simulink model "TrafficLightControl"  (R2020b)
settings: Solver=FixedStepDiscrete  StartTime=0.0  StopTime=150  FixedStep=0.1  RelTol=1e-3  EnableMultiTasking=on
undefined symbols (not defined in the file): DiscIntNeverNeededParam
libraries: simulink x1
settings Model: Creator=baner  LastModifiedBy=baner
settings DataIOCC: ReturnWorkspaceOutputs=off
settings HardwareCC: ProdHWDeviceType=AMD->x86-64 (Windows64)
settings SFSimCC: SimParseCustomCode=off

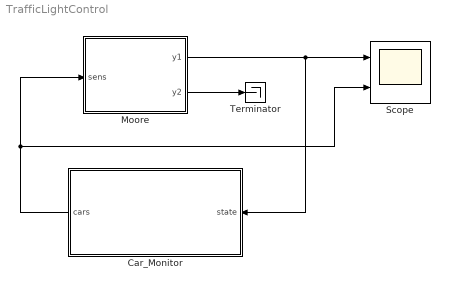
== system TrafficLightControl ==
  Car_Monitor : Subsystem
  Moore : Stateflow chart  TreatAsAtomicUnit=on
  Scope : Scope  NumInputPorts=2
  Terminator : Terminator
  wires:
  Moore/1(y1) -> Car_Monitor/1(state), Scope/1
  Car_Monitor/1(cars) -> Moore/1(sens), Scope/2
  Moore/2(y2) -> Terminator/1

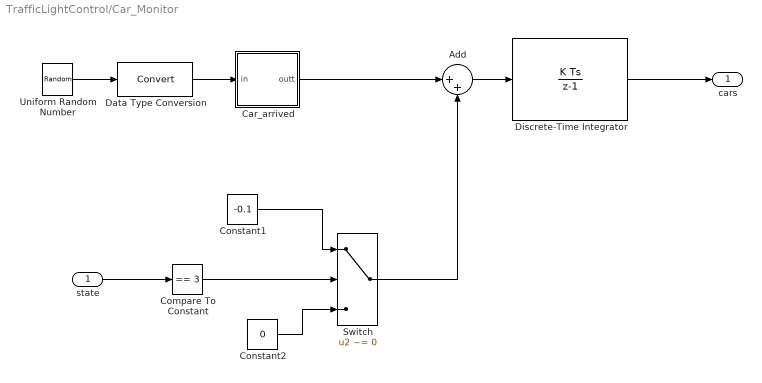
== system TrafficLightControl/Car_Monitor ==
  state : Inport
  Add : Sum  Inputs=|++
  Car_arrived : Stateflow chart  TreatAsAtomicUnit=on
  Compare To Constant : simulink/Logic and Bit Operations/Compare To Constant  relop===  const=3  OutDataTypeStr=boolean  ZeroCross=off
  Constant1 : Constant  Value=-0.1
  Constant2 : Constant  Value=0
  Data Type Conversion : DataTypeConversion
  Discrete-Time Integrator : DiscreteIntegrator  SampleTime=-1  LimitOutput=on  LowerSaturationLimit=0  ICPrevOutput=DiscIntNeverNeededParam  ICPrevScaledInput=DiscIntNeverNeededParam
  Switch : Switch  Criteria=u2 ~= 0
  Uniform Random Number : UniformRandomNumber  Minimum=0  Maximum=100  Seed=177836  SampleTime=0
  cars : Outport  VectorParamsAs1DForOutWhenUnconnected=off
  wires:
  Uniform Random Number/1 -> Data Type Conversion/1
  Data Type Conversion/1 -> Car_arrived/1(in)
  Car_arrived/1(outt) -> Add/1
  Add/1 -> Discrete-Time Integrator/1
  Switch/1 -> Add/2
  Compare To Constant/1 -> Switch/2
  state/1 -> Compare To Constant/1
  Discrete-Time Integrator/1 -> cars/1
  Constant2/1 -> Switch/3
  Constant1/1 -> Switch/1

== stateflow chart TrafficLightControl/Moore ==
  settings: stateMachineType=MOORE_MACHINE  executeAtInitialization=1  initializeOutput=1
  state Stop
    y1 = RED;
    y2 = GREEN;
  state StopForTraffic
    y1 = RED;
    y2 = GREEN;
  state StopToGo
    y1 = RED;
    y2 = YELLOW;
  state Go
    y1 = GREEN;
    y2 = RED;
  state GoToStop
    y1 = YELLOW;
    y2 = RED;
  (default) -> Stop
  StopForTraffic -> StopToGo : [sens]
  Stop -> StopForTraffic : after(20,tick)
  GoToStop -> Stop : after (3,tick)
  StopToGo -> Go : after(3,tick)
  Go -> GoToStop : after(10,tick)
  data: sens input double; y1 output double; RED constant uint8 =1; YELLOW constant double =2; GREEN constant double =3; y2 output double

== stateflow chart TrafficLightControl/Car_Monitor/Car_arrived ==
  (default) -> (junction 2) : {outt = in > 98;}
  data: in input int8; outt output double
